simulink model "MIT_bus_ver3"  (Simulink 8.8)
settings: Solver=VariableStepAuto  StartTime=0.0  StopTime=10.0  RelTol=1e-3
libraries: powerlib x94
settings Model: Creator=jherna4  LastModifiedBy=jherna4
settings DataIOCC: LimitDataPoints=off  SaveFormat=Dataset  SignalLoggingSaveFormat=Dataset
settings DebuggingCC: UnderspecifiedInitializationDetection=Simplified  MergeDetectMultiDrivingBlocksExec=error  FcnCallInpInsideContextMsg=error  StateNameClashWarn=none  SFUnexpectedBacktrackingDiag=error  SFNoUnconditionalDefaultTransitionDiag=error
settings HardwareCC: ProdBitPerPointer=64  ProdBitPerSizeT=64  ProdBitPerPtrDiffT=64  ProdLargestAtomicFloat=Float  ProdIntDivRoundTo=Zero  ProdEndianess=LittleEndian  ProdWordSize=64  ProdHWDeviceType=Intel->x86-64 (Windows64)
settings ModelReferenceCC: PropagateSignalLabelsOutOfModel=on
settings GRTTargetCC: TargetLangStandard=C99 (ISO)  GeneratePreprocessorConditionals=Use local settings  CombineOutputUpdateFcns=on  GRTInterface=off
settings ConfigComp: CovMetricSettings=dwe  CovHtmlReporting=off  CovSaveCumulativeToWorkspaceVar=off  CovSaveSingleToWorkspaceVar=off  CovExternalEMLEnable=on

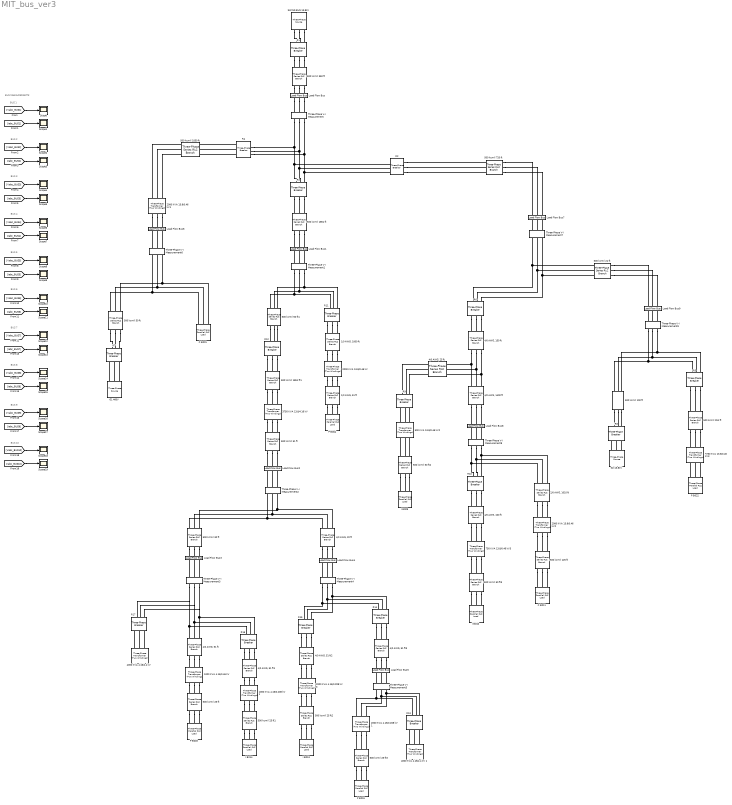
== system MIT_bus_ver3 ==
  note: BUS MEASUREMENTS:
  note: BUS 1
  note: BUS 2
  note: BUS 3
  note: BUS 4
  note: BUS 5
  note: BUS 6
  note: BUS 7
  note: BUS 8
  note: BUS 9
  note: BUS 10
  "1/0 AWG, 1000 ft" : powerlib/Elements/Three-Phase Series RLC Branch  LConnTagsString=A|B|C  RConnTagsString=A|B|C  BranchType=RL  Resistance=128e-3  Inductance=109.81e-6  Measurements=None
  "1/0 AWG, 51 ft" : powerlib/Elements/Three-Phase Series RLC Branch  LConnTagsString=A|B|C  RConnTagsString=A|B|C  BranchType=RL  Resistance=6.53e-3  Inductance=5.6e-6  Measurements=None
  1000 KVA 4.16/0.208 kV 1 : powerlib/Elements/Three-Phase Transformer (Two Windings)  Winding1Connection=Yg  Winding2Connection=Yg  CoreType=Three single-phase transformers  SetSaturation=off  Hysteresis=off  DataFile='hysteresis'  SetInitialFlux=off  Measurements=None  UNITS=pu  NominalPower=[ 1000e3 , 60 ]  Winding1=[4.16e3 0.011 0.02]  Winding2=[0.208e3 0 0]  Rm=500  Lm=500  L0=0.5  Saturation=[0 0;0.0024 1.2;1 1.52]  InitialFluxes=[0.8 -0.8 0.7]  MoreParameters=off  BreakLoop=off  DataType=off  TransfoNumber=1
  "1000 KVA 4.16/0.46 kV " : powerlib/Elements/Three-Phase Transformer (Two Windings)  Winding1Connection=Yg  Winding2Connection=Yg  CoreType=Three single-phase transformers  SetSaturation=off  Hysteresis=off  DataFile='hysteresis'  SetInitialFlux=off  Measurements=None  UNITS=pu  NominalPower=[ 1000e3 , 60 ]  Winding1=[4.16e3 0.011 0.02]  Winding2=[0.46e3 0 0]  Rm=500  Lm=500  L0=0.5  Saturation=[0 0;0.0024 1.2;1 1.52]  InitialFluxes=[0.8 -0.8 0.7]  MoreParameters=off  BreakLoop=off  DataType=off  TransfoNumber=1
  "2/0 AWG, 1010 ft" : powerlib/Elements/Three-Phase Series RLC Branch  LConnTagsString=A|B|C  RConnTagsString=A|B|C  BranchType=RL  Resistance=103e-3  Inductance=109e-6  Measurements=None
  2000 KVA 13.8/0.46 kV : powerlib/Elements/Three-Phase Transformer (Two Windings)  Winding1Connection=Yg  Winding2Connection=Yg  CoreType=Three single-phase transformers  SetSaturation=off  Hysteresis=off  DataFile='hysteresis'  SetInitialFlux=off  Measurements=None  UNITS=pu  NominalPower=[ 2000e3 , 60 ]  Winding1=[13.8e3 0.011 0.02]  Winding2=[0.46e3 0 0]  Rm=500  Lm=500  L0=0.5  Saturation=[0 0;0.0024 1.2;1 1.52]  InitialFluxes=[0.8 -0.8 0.7]  MoreParameters=off  BreakLoop=off  DataType=off  TransfoNumber=1
  2000 KVA 13.8/0.46 kV1 : powerlib/Elements/Three-Phase Transformer (Two Windings)  Winding1Connection=Yg  Winding2Connection=Yg  CoreType=Three single-phase transformers  SetSaturation=off  Hysteresis=off  DataFile='hysteresis'  SetInitialFlux=off  Measurements=None  UNITS=pu  NominalPower=[ 2000e3 , 60 ]  Winding1=[13.8e3 0.011 0.02]  Winding2=[460 0 0]  Rm=500  Lm=500  L0=0.5  Saturation=[0 0;0.0024 1.2;1 1.52]  InitialFluxes=[0.8 -0.8 0.7]  MoreParameters=off  BreakLoop=off  DataType=off  TransfoNumber=1
  2000 KVA 13.8/0.46 kV2 : powerlib/Elements/Three-Phase Transformer (Two Windings)  Winding1Connection=Yg  Winding2Connection=Yg  CoreType=Three single-phase transformers  SetSaturation=off  Hysteresis=off  DataFile='hysteresis'  SetInitialFlux=off  Measurements=None  UNITS=pu  NominalPower=[ 2000e3 , 60 ]  Winding1=[13.8e3 0.011 0.02]  Winding2=[0.46e3 0 0]  Rm=500  Lm=500  L0=0.5  Saturation=[0 0;0.0024 1.2;1 1.52]  InitialFluxes=[0.8 -0.8 0.7]  MoreParameters=off  BreakLoop=off  DataType=off  TransfoNumber=1
  2000 KVA 4.16/0.208 kV 1 : powerlib/Elements/Three-Phase Transformer (Two Windings)  Winding1Connection=Yg  Winding2Connection=Yg  CoreType=Three single-phase transformers  SetSaturation=off  Hysteresis=off  DataFile='hysteresis'  SetInitialFlux=off  Measurements=None  UNITS=pu  NominalPower=[ 2000e3 , 60 ]  Winding1=[4.16e3 0.011 0.02]  Winding2=[0.208e3 0 0]  Rm=500  Lm=500  L0=0.5  Saturation=[0 0;0.0024 1.2;1 1.52]  InitialFluxes=[0.8 -0.8 0.7]  MoreParameters=off  BreakLoop=off  DataType=off  TransfoNumber=1
  2000 KVA 4.16/0.208 kV 3 : powerlib/Elements/Three-Phase Transformer (Two Windings)  Winding1Connection=Yg  Winding2Connection=Yg  CoreType=Three single-phase transformers  SetSaturation=off  Hysteresis=off  DataFile='hysteresis'  SetInitialFlux=off  Measurements=None  UNITS=pu  NominalPower=[ 2000e3 , 60 ]  Winding1=[4.16e3 0.011 0.02]  Winding2=[0.208e3 0 0]  Rm=500  Lm=500  L0=0.5  Saturation=[0 0;0.0024 1.2;1 1.52]  InitialFluxes=[0.8 -0.8 0.7]  MoreParameters=off  BreakLoop=off  DataType=off  TransfoNumber=1
  3750 KVA 13.8/0.46 kV3 : powerlib/Elements/Three-Phase Transformer (Two Windings)  Winding1Connection=Yg  Winding2Connection=Yg  CoreType=Three single-phase transformers  SetSaturation=off  Hysteresis=off  DataFile='hysteresis'  SetInitialFlux=off  Measurements=None  UNITS=pu  NominalPower=[ 3750e3 , 60 ]  Winding1=[13.8e3 0.011 0.02]  Winding2=[0.46e3 0 0]  Rm=500  Lm=500  L0=0.5  Saturation=[0 0;0.0024 1.2;1 1.52]  InitialFluxes=[0.8 -0.8 0.7]  MoreParameters=off  BreakLoop=off  DataType=off  TransfoNumber=1
  "3750 KVA 13.8/4.16 kV " : powerlib/Elements/Three-Phase Transformer (Two Windings)  Winding1Connection=Yg  Winding2Connection=Yg  CoreType=Three single-phase transformers  SetSaturation=off  Hysteresis=off  DataFile='hysteresis'  SetInitialFlux=off  Measurements=None  UNITS=pu  NominalPower=[ 3750e3 , 60 ]  Winding1=[13.8e3 0.011 0.02]  Winding2=[4.16e3 0 0]  Rm=500  Lm=500  L0=0.5  Saturation=[0 0;0.0024 1.2;1 1.52]  InitialFluxes=[0.8 -0.8 0.7]  MoreParameters=off  BreakLoop=off  DataType=off  TransfoNumber=1
  "4/0 AWG, 100 ft" : powerlib/Elements/Three-Phase Series RLC Branch  LConnTagsString=A|B|C  RConnTagsString=A|B|C  BranchType=RL  Resistance=6.4e-3  Inductance=10.11e-6  Measurements=None
  "4/0 AWG, 1400 ft" : powerlib/Elements/Three-Phase Series RLC Branch  LConnTagsString=A|B|C  RConnTagsString=A|B|C  BranchType=RL  Resistance=89.6e-3  Inductance=141.5e-6  Measurements=None
  "4/0 AWG, 150 ft" : powerlib/Elements/Three-Phase Series RLC Branch  LConnTagsString=A|B|C  RConnTagsString=A|B|C  BranchType=RL  Resistance=9.6e-3  Inductance=15.16e-6  Measurements=None
  "4/0 AWG, 20 ft" : powerlib/Elements/Three-Phase Series RLC Branch  LConnTagsString=A|B|C  RConnTagsString=A|B|C  BranchType=RL  Resistance=1.28e-3  Inductance=2.02e-6  Measurements=None
  "4/0 AWG, 25 ft" : powerlib/Elements/Three-Phase Series RLC Branch  LConnTagsString=A|B|C  RConnTagsString=A|B|C  BranchType=RL  Resistance=1.6e-3  Inductance=2.53e-6  Measurements=None
  4/0 AWG, 51 ft{,1..3} (4 alike) : powerlib/Elements/Three-Phase Series RLC Branch  LConnTagsString=A|B|C  RConnTagsString=A|B|C  BranchType=RL  Resistance=3.264e-3  Inductance=5.15e-6  Measurements=None
  4000 KVA 4.16/2.4 kV : powerlib/Elements/Three-Phase Transformer (Two Windings)  Winding1Connection=Yg  Winding2Connection=Yg  CoreType=Three single-phase transformers  SetSaturation=off  Hysteresis=off  DataFile='hysteresis'  SetInitialFlux=off  Measurements=None  UNITS=pu  NominalPower=[ 4000e3 , 60 ]  Winding1=[4160 0.011 0.02]  Winding2=[2400 0 0]  Rm=500  Lm=500  L0=0.5  Saturation=[0 0;0.0024 1.2;1 1.52]  InitialFluxes=[0.8 -0.8 0.7]  MoreParameters=off  BreakLoop=off  DataType=off  TransfoNumber=1
  4000 KVA 4.16/2.4 kV 1 : powerlib/Elements/Three-Phase Transformer (Two Windings)  Winding1Connection=Yg  Winding2Connection=Yg  CoreType=Three single-phase transformers  SetSaturation=off  Hysteresis=off  DataFile='hysteresis'  SetInitialFlux=off  Measurements=None  UNITS=pu  NominalPower=[ 4000e3 , 60 ]  Winding1=[4.16e3 0.011 0.02]  Winding2=[2.4e3 0 0]  Rm=500  Lm=500  L0=0.5  Saturation=[0 0;0.0024 1.2;1 1.52]  InitialFluxes=[0.8 -0.8 0.7]  MoreParameters=off  BreakLoop=off  DataType=off  TransfoNumber=1
  500 KVA 13.8/0.46 kV2 : powerlib/Elements/Three-Phase Transformer (Two Windings)  Winding1Connection=Yg  Winding2Connection=Yg  CoreType=Three single-phase transformers  SetSaturation=off  Hysteresis=off  DataFile='hysteresis'  SetInitialFlux=off  Measurements=None  UNITS=pu  NominalPower=[ 500e3 , 60 ]  Winding1=[13.8e3 0.011 0.02]  Winding2=[0.46e3 0 0]  Rm=500  Lm=500  L0=0.5  Saturation=[0 0;0.0024 1.2;1 1.52]  InitialFluxes=[0.8 -0.8 0.7]  MoreParameters=off  BreakLoop=off  DataType=off  TransfoNumber=1
  500 kcmil 100 ft : powerlib/Elements/Three-Phase Series RLC Branch  LConnTagsString=A|B|C  RConnTagsString=A|B|C  BranchType=RL  Resistance=2.94e-3  Inductance=9.26e-6  Measurements=None
  500 kcmil 1050 ft : powerlib/Elements/Three-Phase Series RLC Branch  LConnTagsString=A|B|C  RConnTagsString=A|B|C  BranchType=RL  Resistance=30.87e-3  Inductance=97.2e-6  Measurements=None
  500 kcmil 125 ft : powerlib/Elements/Three-Phase Series RLC Branch  LConnTagsString=A|B|C  RConnTagsString=A|B|C  BranchType=RL  Resistance=3.7e-3  Inductance=11.6e-6  Measurements=None
  500 kcmil 1851 ft : powerlib/Elements/Three-Phase Series RLC Branch  LConnTagsString=A|B|C  RConnTagsString=A|B|C  BranchType=RL  Resistance=54.41e-3  Inductance=171.36e-6  Measurements=None
  500 kcmil 1851 ft1 : powerlib/Elements/Three-Phase Series RLC Branch  LConnTagsString=A|B|C  RConnTagsString=A|B|C  BranchType=RL  Resistance=54.41e-3  Inductance=171.36e-6  Measurements=None
  500 kcmil 21 ft : powerlib/Elements/Three-Phase Series RLC Branch  LConnTagsString=A|B|C  RConnTagsString=A|B|C  BranchType=RL  Resistance=0.62e-3  Inductance=1.94e-6  Measurements=None
  500 kcmil 25 ft{,1..3} (4 alike) : powerlib/Elements/Three-Phase Series RLC Branch  LConnTagsString=A|B|C  RConnTagsString=A|B|C  BranchType=RL  Resistance=0.735e-3  Inductance=2.31e-6  Measurements=None
  500 kcmil 251 ft : powerlib/Elements/Three-Phase Series RLC Branch  LConnTagsString=A|B|C  RConnTagsString=A|B|C  BranchType=RL  Resistance=7.38e-3  Inductance=23.24e-6  Measurements=None
  500 kcmil 30 ft : powerlib/Elements/Three-Phase Series RLC Branch  LConnTagsString=A|B|C  RConnTagsString=A|B|C  BranchType=RL  Resistance=0.88e-3  Inductance=2.78e-6  Measurements=None
  500 kcmil 350 ft : powerlib/Elements/Three-Phase Series RLC Branch  LConnTagsString=A|B|C  RConnTagsString=A|B|C  BranchType=RL  Resistance=10.29e-3  Inductance=32.4e-6  Measurements=None
  500 kcmil 50 ft{,1..3} (4 alike) : powerlib/Elements/Three-Phase Series RLC Branch  LConnTagsString=A|B|C  RConnTagsString=A|B|C  BranchType=RL  Resistance=1.47e-3  Inductance=4.63e-6  Measurements=None
  500 kcmil 51 ft : powerlib/Elements/Three-Phase Series RLC Branch  LConnTagsString=A|B|C  RConnTagsString=A|B|C  BranchType=RL  Resistance=1.5e-3  Inductance=4.72e-6  Measurements=None
  500 kcmil 720 ft : powerlib/Elements/Three-Phase Series RLC Branch  LConnTagsString=A|B|C  RConnTagsString=A|B|C  BranchType=RL  Resistance=21.17e-3  Inductance=66.65e-6  Measurements=None
  750 KVA 13.8/0.46 kV3 : powerlib/Elements/Three-Phase Transformer (Two Windings)  Winding1Connection=Yg  Winding2Connection=Yg  CoreType=Three single-phase transformers  SetSaturation=off  Hysteresis=off  DataFile='hysteresis'  SetInitialFlux=off  Measurements=None  UNITS=pu  NominalPower=[ 750e3 , 60 ]  Winding1=[13.8e3 0.011 0.02]  Winding2=[0.46e3 0 0]  Rm=500  Lm=500  L0=0.5  Saturation=[0 0;0.0024 1.2;1 1.52]  InitialFluxes=[0.8 -0.8 0.7]  MoreParameters=off  BreakLoop=off  DataType=off  TransfoNumber=1
  C B001 : powerlib/Elements/Three-Phase Parallel RLC Load  LConnTagsString=A|B|C  Configuration=Y (grounded)  NominalVoltage=460  Vabc=[1e3 1e3 1e3]  Vabcp=[1e3 1e3 1e3]  NominalFrequency=60  UnbalancedPower=off  ActivePower=10e3  InductivePower=100  CapacitivePower=100  Pabc=[10e3 9e3 11e3]  QLabc=[100 90 110]  QCabc=[100 90 110]  Pabcp=[10e3 9e3 11e3]  QLabcp=[100 90 110]  QCabcp=[100 90 110]  Measurements=None  LoadType=constant Z
  C B011 : powerlib/Elements/Three-Phase Parallel RLC Load  LConnTagsString=A|B|C  Configuration=Y (grounded)  NominalVoltage=460  Vabc=[1e3 1e3 1e3]  Vabcp=[1e3 1e3 1e3]  NominalFrequency=60  UnbalancedPower=off  ActivePower=10e3  InductivePower=100  CapacitivePower=100  Pabc=[10e3 9e3 11e3]  QLabc=[100 90 110]  QCabc=[100 90 110]  Pabcp=[10e3 9e3 11e3]  QLabcp=[100 90 110]  QCabcp=[100 90 110]  Measurements=None  LoadType=constant Z
  G1 460V : powerlib/Electrical Sources/Three-Phase Source  InternalConnection=Yg  VoltagePhases=on  Voltage=120e3  PhaseAngle=0  Voltage_phases=[1 1 1]*460/sqrt(3)  PhaseAngles_phases=[ 0 -120 120]  Frequency=60  NonIdealSource=off  SpecifyImpedance=on  Resistance=0.8929  Inductance=16.58e-3  ShortCircuitLevel=100e6  BaseVoltage=120e3  XRratio=10  BusType=swing  Pref=0  Qref=0  Prefabc=[0 0 0]  Qrefabc=[0 0 0]  Qmin="[-inf  -inf -inf]"  Qmax="[inf  inf inf]"
  G2 13.8kV : powerlib/Electrical Sources/Three-Phase Source  InternalConnection=Yg  VoltagePhases=on  Voltage=120e3  PhaseAngle=0  Voltage_phases=[1 1 1]*13.8e3/sqrt(3)  PhaseAngles_phases=[ 0 -120 120]  Frequency=60  NonIdealSource=off  SpecifyImpedance=on  Resistance=0.8929  Inductance=16.58e-3  ShortCircuitLevel=100e6  BaseVoltage=120e3  XRratio=10  BusType=swing  Pref=0  Qref=0  Prefabc=[0 0 0]  Qrefabc=[0 0 0]  Qmin="[-inf  -inf -inf]"  Qmax="[inf  inf inf]"
  I B009 : powerlib/Elements/Three-Phase Parallel RLC Load  LConnTagsString=A|B|C  Configuration=Y (grounded)  NominalVoltage=460  Vabc=[1e3 1e3 1e3]  Vabcp=[1e3 1e3 1e3]  NominalFrequency=60  UnbalancedPower=off  ActivePower=10e3  InductivePower=100  CapacitivePower=100  Pabc=[10e3 9e3 11e3]  QLabc=[100 90 110]  QCabc=[100 90 110]  Pabcp=[10e3 9e3 11e3]  QLabcp=[100 90 110]  QCabcp=[100 90 110]  Measurements=None  LoadType=constant Z
  I B010 : powerlib/Elements/Three-Phase Parallel RLC Load  LConnTagsString=A|B|C  Configuration=Y (grounded)  NominalVoltage=460  Vabc=[1e3 1e3 1e3]  Vabcp=[1e3 1e3 1e3]  NominalFrequency=60  UnbalancedPower=off  ActivePower=10e3  InductivePower=100  CapacitivePower=100  Pabc=[10e3 9e3 11e3]  QLabc=[100 90 110]  QCabc=[100 90 110]  Pabcp=[10e3 9e3 11e3]  QLabcp=[100 90 110]  QCabcp=[100 90 110]  Measurements=None  LoadType=constant Z
  I B013 : powerlib/Elements/Three-Phase Parallel RLC Load  LConnTagsString=A|B|C  Configuration=Y (grounded)  NominalVoltage=208  Vabc=[1e3 1e3 1e3]  Vabcp=[1e3 1e3 1e3]  NominalFrequency=60  UnbalancedPower=off  ActivePower=10e3  InductivePower=100  CapacitivePower=100  Pabc=[10e3 9e3 11e3]  QLabc=[100 90 110]  QCabc=[100 90 110]  Pabcp=[10e3 9e3 11e3]  QLabcp=[100 90 110]  QCabcp=[100 90 110]  Measurements=None  LoadType=constant Z
  I B014 : powerlib/Elements/Three-Phase Parallel RLC Load  LConnTagsString=A|B|C  Configuration=Y (grounded)  NominalVoltage=208  Vabc=[1e3 1e3 1e3]  Vabcp=[1e3 1e3 1e3]  NominalFrequency=60  UnbalancedPower=off  ActivePower=10e3  InductivePower=100  CapacitivePower=100  Pabc=[10e3 9e3 11e3]  QLabc=[100 90 110]  QCabc=[100 90 110]  Pabcp=[10e3 9e3 11e3]  QLabcp=[100 90 110]  QCabcp=[100 90 110]  Measurements=None  LoadType=constant Z
  Load Flow Bus : powerlib/Measurements/Load Flow Bus  LConnTagsString=a|b|c  RConnTagsString=a|b|c  Phases=ABC  Connectors=on both sides  ID=BUS1  Vbase=13.8e3/sqrt(3)  Vref=[1 1 1]  Vangle=[0 -120 120]  VLF=1  VLFb=1  VLFc=1  angleLF=0  angleLFb=0  angleLFc=0
  Load Flow Bus1 : powerlib/Measurements/Load Flow Bus  LConnTagsString=a|b|c  RConnTagsString=a|b|c  Phases=ABC  Connectors=on both sides  ID=BUS3  Vbase=13.8e3/sqrt(3)  Vref=[1 1 1]  Vangle=[1 -120 120]  VLF=1  VLFb=1  VLFc=1  angleLF=0  angleLFb=0  angleLFc=0
  Load Flow Bus2 : powerlib/Measurements/Load Flow Bus  LConnTagsString=a|b|c  RConnTagsString=a|b|c  Phases=ABC  Connectors=on both sides  ID=BUS4  Vbase=4.16e3/sqrt(3)  Vref=[1 1 1]  Vangle=[0 -120 120]  VLF=1  VLFb=1  VLFc=1  angleLF=0  angleLFb=0  angleLFc=0
  Load Flow Bus3 : powerlib/Measurements/Load Flow Bus  LConnTagsString=a|b|c  RConnTagsString=a|b|c  Phases=ABC  Connectors=on both sides  ID=BUS5  Vbase=4.16e3/sqrt(3)  Vref=[1 1 1]  Vangle=[0 -120 120]  VLF=1  VLFb=1  VLFc=1  angleLF=0  angleLFb=0  angleLFc=0
  Load Flow Bus4 : powerlib/Measurements/Load Flow Bus  LConnTagsString=a|b|c  RConnTagsString=a|b|c  Phases=ABC  Connectors=on both sides  ID=BUS6  Vbase=4.16e3/sqrt(3)  Vref=[1 1 1]  Vangle=[0 -120 120]  VLF=1  VLFb=1  VLFc=1  angleLF=0  angleLFb=0  angleLFc=0
  Load Flow Bus5 : powerlib/Measurements/Load Flow Bus  LConnTagsString=a|b|c  RConnTagsString=a|b|c  Phases=ABC  Connectors=on both sides  ID=BUS7  Vbase=4.16e3/sqrt(3)  Vref=[1 1 1]  Vangle=[0 -120 120]  VLF=1  VLFb=1  VLFc=1  angleLF=0  angleLFb=0  angleLFc=0
  Load Flow Bus6 : powerlib/Measurements/Load Flow Bus  LConnTagsString=a|b|c  RConnTagsString=a|b|c  Phases=ABC  Connectors=on both sides  ID=BUS2  Vbase=460/sqrt(3)  Vref=[1 1 1]  Vangle=[0 -120 120]  VLF=1  VLFb=1  VLFc=1  angleLF=0  angleLFb=0  angleLFc=0
  Load Flow Bus7 : powerlib/Measurements/Load Flow Bus  LConnTagsString=a|b|c  RConnTagsString=a|b|c  Phases=ABC  Connectors=on both sides  ID=BUS8  Vbase=13.8e3/sqrt(3)  Vref=[1 1 1]  Vangle=[0 -120 120]  VLF=1  VLFb=1  VLFc=1  angleLF=0  angleLFb=0  angleLFc=0
  Load Flow Bus8 : powerlib/Measurements/Load Flow Bus  LConnTagsString=a|b|c  RConnTagsString=a|b|c  Phases=ABC  Connectors=on both sides  ID=BUS9  Vbase=13.8e3/sqrt(3)  Vref=[1 1 1]  Vangle=[0 -120 120]  VLF=1  VLFb=1  VLFc=1  angleLF=0  angleLFb=0  angleLFc=0
  Load Flow Bus9 : powerlib/Measurements/Load Flow Bus  LConnTagsString=a|b|c  RConnTagsString=a|b|c  Phases=ABC  Connectors=on both sides  ID=BUS10  Vbase=13.8e3/sqrt(3)  Vref=[1 1 1]  Vangle=[0 -120 120]  VLF=1  VLFb=1  VLFc=1  angleLF=0  angleLFb=0  angleLFc=0
  P B003 : powerlib/Elements/Three-Phase Parallel RLC Load  LConnTagsString=A|B|C  Configuration=Y (grounded)  NominalVoltage=460  Vabc=[1e3 1e3 1e3]  Vabcp=[1e3 1e3 1e3]  NominalFrequency=60  UnbalancedPower=off  ActivePower=10e3  InductivePower=100  CapacitivePower=100  Pabc=[10e3 9e3 11e3]  QLabc=[100 90 110]  QCabc=[100 90 110]  Pabcp=[10e3 9e3 11e3]  QLabcp=[100 90 110]  QCabcp=[100 90 110]  Measurements=None  LoadType=constant Z
  P B004 : powerlib/Elements/Three-Phase Parallel RLC Load  LConnTagsString=A|B|C  Configuration=Y (grounded)  NominalVoltage=460  Vabc=[1e3 1e3 1e3]  Vabcp=[1e3 1e3 1e3]  NominalFrequency=60  UnbalancedPower=off  ActivePower=10e3  InductivePower=100  CapacitivePower=100  Pabc=[10e3 9e3 11e3]  QLabc=[100 90 110]  QCabc=[100 90 110]  Pabcp=[10e3 9e3 11e3]  QLabcp=[100 90 110]  QCabcp=[100 90 110]  Measurements=None  LoadType=constant Z
  P B015 : powerlib/Elements/Three-Phase Parallel RLC Load  LConnTagsString=A|B|C  Configuration=Y (grounded)  NominalVoltage=208  Vabc=[1e3 1e3 1e3]  Vabcp=[1e3 1e3 1e3]  NominalFrequency=60  UnbalancedPower=off  ActivePower=10e3  InductivePower=100  CapacitivePower=100  Pabc=[10e3 9e3 11e3]  QLabc=[100 90 110]  QCabc=[100 90 110]  Pabcp=[10e3 9e3 11e3]  QLabcp=[100 90 110]  QCabcp=[100 90 110]  Measurements=None  LoadType=constant Z
  P B022 : powerlib/Elements/Three-Phase Parallel RLC Load  LConnTagsString=A|B|C  Configuration=Y (grounded)  NominalVoltage=460  Vabc=[1e3 1e3 1e3]  Vabcp=[1e3 1e3 1e3]  NominalFrequency=60  UnbalancedPower=off  ActivePower=10e3  InductivePower=100  CapacitivePower=100  Pabc=[10e3 9e3 11e3]  QLabc=[100 90 110]  QCabc=[100 90 110]  Pabcp=[10e3 9e3 11e3]  QLabcp=[100 90 110]  QCabcp=[100 90 110]  Measurements=None  LoadType=constant Z
  R{1..17} (17 alike) : powerlib/Elements/Three-Phase Breaker  InitialState=closed  SwitchA=off  SwitchB=off  SwitchC=off  SwitchTimes=[0.5 ]  External=on  BreakerResistance=0.0001  SnubberResistance=inf  SnubberCapacitance=0  Measurements=None
  "SWING BUS 13.8kV " : powerlib/Electrical Sources/Three-Phase Source  InternalConnection=Yg  VoltagePhases=on  Voltage=120e3  PhaseAngle=0  Voltage_phases=[1 1 1]*13.8e3/sqrt(3)  PhaseAngles_phases=[ 0 -120 120]  Frequency=60  NonIdealSource=off  SpecifyImpedance=on  Resistance=0.8929  Inductance=16.58e-3  ShortCircuitLevel=100e6  BaseVoltage=120e3  XRratio=10  BusType=swing  Pref=0  Qref=0  Prefabc=[0 0 0]  Qrefabc=[0 0 0]  Qmin="[-inf  -inf -inf]"  Qmax="[inf  inf inf]"
  Scope{,1..19} (20 alike) : Scope
  Three-Phase V-I Measurement : powerlib/Measurements/Three-Phase V-I Measurement  VoltageMeasurement=phase-to-ground  SetLabelV=on  LabelV=Vabc_BUS1  Vpu=off  VpuLL=off  CurrentMeasurement=yes  SetLabelI=on  LabelI=Iabc_BUS1  Ipu=off  Pbase=100e6  Vbase=500e3  OutputType=Complex  PhasorSimulation=off  PSBequivalent=0
  Three-Phase V-I Measurement1 : powerlib/Measurements/Three-Phase V-I Measurement  VoltageMeasurement=phase-to-ground  SetLabelV=on  LabelV=Vabc_BUS3  Vpu=off  VpuLL=off  CurrentMeasurement=yes  SetLabelI=on  LabelI=Iabc_BUS3  Ipu=off  Pbase=100e6  Vbase=500e3  OutputType=Complex  PhasorSimulation=off  PSBequivalent=0
  Three-Phase V-I Measurement2 : powerlib/Measurements/Three-Phase V-I Measurement  VoltageMeasurement=phase-to-ground  SetLabelV=on  LabelV=Vabc_BUS4  Vpu=off  VpuLL=off  CurrentMeasurement=yes  SetLabelI=on  LabelI=Iabc_BUS4  Ipu=off  Pbase=100e6  Vbase=500e3  OutputType=Complex  PhasorSimulation=off  PSBequivalent=0
  Three-Phase V-I Measurement3 : powerlib/Measurements/Three-Phase V-I Measurement  VoltageMeasurement=phase-to-ground  SetLabelV=on  LabelV=Vabc_BUS5  Vpu=off  VpuLL=off  CurrentMeasurement=yes  SetLabelI=on  LabelI=Iabc_BUS5  Ipu=off  Pbase=100e6  Vbase=500e3  OutputType=Complex  PhasorSimulation=off  PSBequivalent=0
  Three-Phase V-I Measurement4 : powerlib/Measurements/Three-Phase V-I Measurement  VoltageMeasurement=phase-to-ground  SetLabelV=on  LabelV=Vabc_BUS6  Vpu=off  VpuLL=off  CurrentMeasurement=yes  SetLabelI=on  LabelI=Iabc_BUS6  Ipu=off  Pbase=100e6  Vbase=500e3  OutputType=Complex  PhasorSimulation=off  PSBequivalent=0
  Three-Phase V-I Measurement5 : powerlib/Measurements/Three-Phase V-I Measurement  VoltageMeasurement=phase-to-ground  SetLabelV=on  LabelV=Vabc_BUS7  Vpu=off  VpuLL=off  CurrentMeasurement=yes  SetLabelI=on  LabelI=Iabc_BUS7  Ipu=off  Pbase=100e6  Vbase=500e3  OutputType=Complex  PhasorSimulation=off  PSBequivalent=0
  Three-Phase V-I Measurement6 : powerlib/Measurements/Three-Phase V-I Measurement  VoltageMeasurement=phase-to-ground  SetLabelV=on  LabelV=Vabc_BUS2  Vpu=off  VpuLL=off  CurrentMeasurement=yes  SetLabelI=on  LabelI=Iabc_BUS2  Ipu=off  Pbase=100e6  Vbase=500e3  OutputType=Complex  PhasorSimulation=off  PSBequivalent=0
  Three-Phase V-I Measurement7 : powerlib/Measurements/Three-Phase V-I Measurement  VoltageMeasurement=phase-to-ground  SetLabelV=on  LabelV=Vabc_BUS8  Vpu=off  VpuLL=off  CurrentMeasurement=yes  SetLabelI=on  LabelI=Iabc_BUS8  Ipu=off  Pbase=100e6  Vbase=500e3  OutputType=Complex  PhasorSimulation=off  PSBequivalent=0
  Three-Phase V-I Measurement8 : powerlib/Measurements/Three-Phase V-I Measurement  VoltageMeasurement=phase-to-ground  SetLabelV=on  LabelV=Vabc_BUS9  Vpu=off  VpuLL=off  CurrentMeasurement=yes  SetLabelI=on  LabelI=Iabc_BUS9  Ipu=off  Pbase=100e6  Vbase=500e3  OutputType=Complex  PhasorSimulation=off  PSBequivalent=0
  Three-Phase V-I Measurement9 : powerlib/Measurements/Three-Phase V-I Measurement  VoltageMeasurement=phase-to-ground  SetLabelV=on  LabelV=Vabc_BUS10  Vpu=off  VpuLL=off  CurrentMeasurement=yes  SetLabelI=on  LabelI=Iabc_BUS10  Ipu=off  Pbase=100e6  Vbase=500e3  OutputType=Complex  PhasorSimulation=off  PSBequivalent=0
  wires:
  [Vabc_BUS1] -> Scope/1
  [Iabc_BUS1] -> Scope1/1
  [Vabc_BUS2] -> Scope2/1
  [Iabc_BUS2] -> Scope3/1
  [Vabc_BUS3] -> Scope4/1
  [Iabc_BUS3] -> Scope5/1
  [Vabc_BUS4] -> Scope6/1
  [Iabc_BUS4] -> Scope7/1
  [Vabc_BUS5] -> Scope8/1
  [Iabc_BUS5] -> Scope9/1
  [Vabc_BUS6] -> Scope10/1
  [Iabc_BUS6] -> Scope11/1
  [Vabc_BUS7] -> Scope12/1
  [Iabc_BUS7] -> Scope13/1
  [Vabc_BUS8] -> Scope14/1
  [Iabc_BUS8] -> Scope15/1
  [Vabc_BUS9] -> Scope16/1
  [Iabc_BUS9] -> Scope17/1
  [Vabc_BUS10] -> Scope18/1
  [Iabc_BUS10] -> Scope19/1
  connections:
  "SWING BUS 13.8kV "/RConn1 -- R1/LConn1
  "SWING BUS 13.8kV "/RConn2 -- R1/LConn2
  "SWING BUS 13.8kV "/RConn3 -- R1/LConn3
  Three-Phase V-I Measurement1/RConn1 -- 500 kcmil 50 ft1/LConn1 -- R11/LConn1
  Three-Phase V-I Measurement1/RConn2 -- 500 kcmil 50 ft1/LConn2 -- R11/LConn2
  Three-Phase V-I Measurement1/RConn3 -- 500 kcmil 50 ft1/LConn3 -- R11/LConn3
  Load Flow Bus/RConn3 -- Three-Phase V-I Measurement/LConn3
  Load Flow Bus/RConn2 -- Three-Phase V-I Measurement/LConn2
  Load Flow Bus/RConn1 -- Three-Phase V-I Measurement/LConn1
  Three-Phase V-I Measurement/RConn3 -- R4/LConn3 -- R2/LConn3 -- R3/LConn3
  Three-Phase V-I Measurement/RConn2 -- R4/LConn2 -- R2/LConn2 -- R3/LConn2
  Three-Phase V-I Measurement/RConn1 -- R4/LConn1 -- R2/LConn1 -- R3/LConn1
  Three-Phase V-I Measurement1/LConn1 -- Load Flow Bus1/RConn1
  Three-Phase V-I Measurement1/LConn2 -- Load Flow Bus1/RConn2
  Three-Phase V-I Measurement1/LConn3 -- Load Flow Bus1/RConn3
  Three-Phase V-I Measurement2/LConn3 -- Load Flow Bus2/RConn3
  Three-Phase V-I Measurement2/LConn2 -- Load Flow Bus2/RConn2
  Three-Phase V-I Measurement2/LConn1 -- Load Flow Bus2/RConn1
  Three-Phase V-I Measurement3/RConn3 -- R17/LConn3 -- "4/0 AWG, 51 ft"/LConn3 -- R16/LConn3
  Three-Phase V-I Measurement3/RConn2 -- R17/LConn2 -- "4/0 AWG, 51 ft"/LConn2 -- R16/LConn2
  500 kcmil 30 ft/LConn1 -- "4/0 AWG, 20 ft"/LConn1 -- Three-Phase V-I Measurement2/RConn1
  4000 KVA 4.16/2.4 kV/LConn3 -- R17/RConn3
  4000 KVA 4.16/2.4 kV/LConn2 -- R17/RConn2
  4000 KVA 4.16/2.4 kV/LConn1 -- R17/RConn1
  Three-Phase V-I Measurement5/LConn2 -- Load Flow Bus5/RConn2
  Three-Phase V-I Measurement5/LConn1 -- Load Flow Bus5/RConn1
  Three-Phase V-I Measurement5/LConn3 -- Load Flow Bus5/RConn3
  2000 KVA 4.16/0.208 kV 1/LConn1 -- R13/LConn1 -- Three-Phase V-I Measurement5/RConn1
  2000 KVA 4.16/0.208 kV 1/LConn2 -- R13/LConn2 -- Three-Phase V-I Measurement5/RConn2
  2000 KVA 4.16/0.208 kV 1/LConn3 -- R13/LConn3 -- Three-Phase V-I Measurement5/RConn3
  4000 KVA 4.16/2.4 kV 1/LConn1 -- R13/RConn1
  4000 KVA 4.16/2.4 kV 1/LConn2 -- R13/RConn2
  4000 KVA 4.16/2.4 kV 1/LConn3 -- R13/RConn3
  500 kcmil 1050 ft/RConn3 -- 2000 KVA 13.8/0.46 kV1/LConn3
  500 kcmil 1050 ft/RConn2 -- 2000 KVA 13.8/0.46 kV1/LConn2
  500 kcmil 1050 ft/RConn1 -- 2000 KVA 13.8/0.46 kV1/LConn1
  2000 KVA 13.8/0.46 kV1/RConn3 -- Load Flow Bus6/LConn3
  2000 KVA 13.8/0.46 kV1/RConn2 -- Load Flow Bus6/LConn2
  2000 KVA 13.8/0.46 kV1/RConn1 -- Load Flow Bus6/LConn1
  Three-Phase V-I Measurement6/LConn1 -- Load Flow Bus6/RConn1
  Three-Phase V-I Measurement6/LConn2 -- Load Flow Bus6/RConn2
  Three-Phase V-I Measurement6/LConn3 -- Load Flow Bus6/RConn3
  C B001/LConn1 -- 500 kcmil 50 ft/LConn1 -- Three-Phase V-I Measurement6/RConn1
  C B001/LConn2 -- 500 kcmil 50 ft/LConn2 -- Three-Phase V-I Measurement6/RConn2
  C B001/LConn3 -- 500 kcmil 50 ft/LConn3 -- Three-Phase V-I Measurement6/RConn3
  Three-Phase V-I Measurement7/LConn1 -- Load Flow Bus7/RConn1
  Three-Phase V-I Measurement7/LConn3 -- Load Flow Bus7/RConn3
  Three-Phase V-I Measurement7/LConn2 -- Load Flow Bus7/RConn2
  500 KVA 13.8/0.46 kV2/LConn3 -- R9/RConn3
  500 KVA 13.8/0.46 kV2/LConn2 -- R9/RConn2
  500 KVA 13.8/0.46 kV2/LConn1 -- R9/RConn1
  Three-Phase V-I Measurement8/RConn3 -- "2/0 AWG, 1010 ft"/LConn3 -- R10/LConn3
  "4/0 AWG, 150 ft"/RConn1 -- "4/0 AWG, 1400 ft"/LConn1 -- "4/0 AWG, 25 ft"/LConn1
  "4/0 AWG, 150 ft"/RConn2 -- "4/0 AWG, 1400 ft"/LConn2 -- "4/0 AWG, 25 ft"/LConn2
  Three-Phase V-I Measurement9/RConn1 -- 500 kcmil 100 ft/LConn1 -- R5/LConn1
  Three-Phase V-I Measurement9/RConn2 -- 500 kcmil 100 ft/LConn2 -- R5/LConn2
  Three-Phase V-I Measurement9/RConn3 -- 500 kcmil 100 ft/LConn3 -- R5/LConn3
  G1 460V/RConn1 -- R7/RConn1
  G1 460V/RConn2 -- R7/RConn2
  G1 460V/RConn3 -- R7/RConn3
  Three-Phase V-I Measurement3/LConn1 -- Load Flow Bus3/RConn1
  Three-Phase V-I Measurement3/LConn3 -- Load Flow Bus3/RConn3
  Three-Phase V-I Measurement3/LConn2 -- Load Flow Bus3/RConn2
  500 kcmil 30 ft/LConn3 -- "4/0 AWG, 20 ft"/LConn3 -- Three-Phase V-I Measurement2/RConn3
  500 kcmil 30 ft/LConn2 -- "4/0 AWG, 20 ft"/LConn2 -- Three-Phase V-I Measurement2/RConn2
  Three-Phase V-I Measurement3/RConn1 -- R17/LConn1 -- "4/0 AWG, 51 ft"/LConn1 -- R16/LConn1
  Three-Phase V-I Measurement4/LConn3 -- Load Flow Bus4/RConn3
  Three-Phase V-I Measurement4/LConn2 -- Load Flow Bus4/RConn2
  Three-Phase V-I Measurement4/LConn1 -- Load Flow Bus4/RConn1
  R14/LConn1 -- Three-Phase V-I Measurement4/RConn1 -- R15/LConn1
  R14/LConn2 -- Three-Phase V-I Measurement4/RConn2 -- R15/LConn2
  R14/LConn3 -- Three-Phase V-I Measurement4/RConn3 -- R15/LConn3
  Three-Phase V-I Measurement8/LConn3 -- Load Flow Bus8/RConn3
  Three-Phase V-I Measurement8/LConn1 -- Load Flow Bus8/RConn1
  Three-Phase V-I Measurement8/LConn2 -- Load Flow Bus8/RConn2
  "4/0 AWG, 150 ft"/RConn3 -- "4/0 AWG, 1400 ft"/LConn3 -- "4/0 AWG, 25 ft"/LConn3
  Three-Phase V-I Measurement8/RConn2 -- "2/0 AWG, 1010 ft"/LConn2 -- R10/LConn2
  Three-Phase V-I Measurement8/RConn1 -- "2/0 AWG, 1010 ft"/LConn1 -- R10/LConn1
  Three-Phase V-I Measurement9/LConn3 -- Load Flow Bus9/RConn3
  Three-Phase V-I Measurement9/LConn1 -- Load Flow Bus9/RConn1
  Three-Phase V-I Measurement9/LConn2 -- Load Flow Bus9/RConn2
  R6/LConn1 -- 500 kcmil 21 ft/LConn1 -- Three-Phase V-I Measurement7/RConn1
  R6/LConn2 -- 500 kcmil 21 ft/LConn2 -- Three-Phase V-I Measurement7/RConn2
  R6/LConn3 -- 500 kcmil 21 ft/LConn3 -- Three-Phase V-I Measurement7/RConn3
  P B022/LConn3 -- 3750 KVA 13.8/0.46 kV3/RConn3
  P B022/LConn2 -- 3750 KVA 13.8/0.46 kV3/RConn2
  P B022/LConn1 -- 3750 KVA 13.8/0.46 kV3/RConn1
  G2 13.8kV/RConn3 -- R8/RConn3
  G2 13.8kV/RConn2 -- R8/RConn2
  G2 13.8kV/RConn1 -- R8/RConn1
  R1/RConn3 -- 500 kcmil 350 ft/LConn3
  R1/RConn2 -- 500 kcmil 350 ft/LConn2
  R1/RConn1 -- 500 kcmil 350 ft/LConn1
  500 kcmil 350 ft/RConn1 -- Load Flow Bus/LConn1
  500 kcmil 350 ft/RConn2 -- Load Flow Bus/LConn2
  500 kcmil 350 ft/RConn3 -- Load Flow Bus/LConn3
  500 kcmil 50 ft/RConn1 -- R7/LConn1
  500 kcmil 50 ft/RConn2 -- R7/LConn2
  500 kcmil 50 ft/RConn3 -- R7/LConn3
  R3/RConn3 -- 500 kcmil 1851 ft/LConn3
  500 kcmil 1851 ft/RConn3 -- Load Flow Bus1/LConn3
  R3/RConn2 -- 500 kcmil 1851 ft/LConn2
  500 kcmil 1851 ft/RConn2 -- Load Flow Bus1/LConn2
  R3/RConn1 -- 500 kcmil 1851 ft/LConn1
  500 kcmil 1851 ft/RConn1 -- Load Flow Bus1/LConn1
  500 kcmil 50 ft1/RConn3 -- R12/LConn3
  500 kcmil 50 ft1/RConn2 -- R12/LConn2
  500 kcmil 50 ft1/RConn1 -- R12/LConn1
  R12/RConn3 -- 500 kcmil 1851 ft1/LConn3
  500 kcmil 1851 ft1/RConn3 -- "3750 KVA 13.8/4.16 kV "/LConn3
  R12/RConn2 -- 500 kcmil 1851 ft1/LConn2
  500 kcmil 1851 ft1/RConn2 -- "3750 KVA 13.8/4.16 kV "/LConn2
  R12/RConn1 -- 500 kcmil 1851 ft1/LConn1
  500 kcmil 1851 ft1/RConn1 -- "3750 KVA 13.8/4.16 kV "/LConn1
  "3750 KVA 13.8/4.16 kV "/RConn3 -- 500 kcmil 51 ft/LConn3
  "3750 KVA 13.8/4.16 kV "/RConn2 -- 500 kcmil 51 ft/LConn2
  "3750 KVA 13.8/4.16 kV "/RConn1 -- 500 kcmil 51 ft/LConn1
  500 kcmil 51 ft/RConn3 -- Load Flow Bus2/LConn3
  500 kcmil 51 ft/RConn2 -- Load Flow Bus2/LConn2
  500 kcmil 51 ft/RConn1 -- Load Flow Bus2/LConn1
  R11/RConn1 -- "1/0 AWG, 1000 ft"/LConn1
  R11/RConn2 -- "1/0 AWG, 1000 ft"/LConn2
  R11/RConn3 -- "1/0 AWG, 1000 ft"/LConn3
  "1/0 AWG, 1000 ft"/RConn1 -- 2000 KVA 13.8/0.46 kV/LConn1
  "1/0 AWG, 1000 ft"/RConn2 -- 2000 KVA 13.8/0.46 kV/LConn2
  "1/0 AWG, 1000 ft"/RConn3 -- 2000 KVA 13.8/0.46 kV/LConn3
  2000 KVA 13.8/0.46 kV/RConn1 -- "1/0 AWG, 51 ft"/LConn1
  2000 KVA 13.8/0.46 kV/RConn2 -- "1/0 AWG, 51 ft"/LConn2
  2000 KVA 13.8/0.46 kV/RConn3 -- "1/0 AWG, 51 ft"/LConn3
  "1/0 AWG, 51 ft"/RConn1 -- P B004/LConn1
  "1/0 AWG, 51 ft"/RConn2 -- P B004/LConn2
  "1/0 AWG, 51 ft"/RConn3 -- P B004/LConn3
  500 kcmil 30 ft/RConn3 -- Load Flow Bus3/LConn3
  500 kcmil 30 ft/RConn2 -- Load Flow Bus3/LConn2
  500 kcmil 30 ft/RConn1 -- Load Flow Bus3/LConn1
  "4/0 AWG, 20 ft"/RConn3 -- Load Flow Bus4/LConn3
  "4/0 AWG, 20 ft"/RConn2 -- Load Flow Bus4/LConn2
  "4/0 AWG, 20 ft"/RConn1 -- Load Flow Bus4/LConn1
  "4/0 AWG, 51 ft"/RConn3 -- "1000 KVA 4.16/0.46 kV "/LConn3
  "4/0 AWG, 51 ft"/RConn2 -- "1000 KVA 4.16/0.46 kV "/LConn2
  "4/0 AWG, 51 ft"/RConn1 -- "1000 KVA 4.16/0.46 kV "/LConn1
  "1000 KVA 4.16/0.46 kV "/RConn3 -- 500 kcmil 25 ft/LConn3
  "1000 KVA 4.16/0.46 kV "/RConn2 -- 500 kcmil 25 ft/LConn2
  "1000 KVA 4.16/0.46 kV "/RConn1 -- 500 kcmil 25 ft/LConn1
  500 kcmil 25 ft/RConn1 -- P B003/LConn1
  500 kcmil 25 ft/RConn2 -- P B003/LConn2
  500 kcmil 25 ft/RConn3 -- P B003/LConn3
  R16/RConn3 -- "4/0 AWG, 51 ft1"/LConn3
  R16/RConn2 -- "4/0 AWG, 51 ft1"/LConn2
  R16/RConn1 -- "4/0 AWG, 51 ft1"/LConn1
  "4/0 AWG, 51 ft1"/RConn3 -- 1000 KVA 4.16/0.208 kV 1/LConn3
  "4/0 AWG, 51 ft1"/RConn2 -- 1000 KVA 4.16/0.208 kV 1/LConn2
  "4/0 AWG, 51 ft1"/RConn1 -- 1000 KVA 4.16/0.208 kV 1/LConn1
  1000 KVA 4.16/0.208 kV 1/RConn3 -- 500 kcmil 25 ft1/LConn3
  1000 KVA 4.16/0.208 kV 1/RConn2 -- 500 kcmil 25 ft1/LConn2
  1000 KVA 4.16/0.208 kV 1/RConn1 -- 500 kcmil 25 ft1/LConn1
  500 kcmil 25 ft1/RConn3 -- I B014/LConn3
  500 kcmil 25 ft1/RConn2 -- I B014/LConn2
  500 kcmil 25 ft1/RConn1 -- I B014/LConn1
  R15/RConn3 -- "4/0 AWG, 51 ft2"/LConn3
  R15/RConn2 -- "4/0 AWG, 51 ft2"/LConn2
  R15/RConn1 -- "4/0 AWG, 51 ft2"/LConn1
  "4/0 AWG, 51 ft2"/RConn3 -- 2000 KVA 4.16/0.208 kV 3/LConn3
  "4/0 AWG, 51 ft2"/RConn2 -- 2000 KVA 4.16/0.208 kV 3/LConn2
  "4/0 AWG, 51 ft2"/RConn1 -- 2000 KVA 4.16/0.208 kV 3/LConn1
  2000 KVA 4.16/0.208 kV 3/RConn3 -- 500 kcmil 25 ft2/LConn3
  2000 KVA 4.16/0.208 kV 3/RConn2 -- 500 kcmil 25 ft2/LConn2
  2000 KVA 4.16/0.208 kV 3/RConn1 -- 500 kcmil 25 ft2/LConn1
  500 kcmil 25 ft2/RConn1 -- I B013/LConn1
  500 kcmil 25 ft2/RConn2 -- I B013/LConn2
  500 kcmil 25 ft2/RConn3 -- I B013/LConn3
  R14/RConn1 -- "4/0 AWG, 51 ft3"/LConn1
  R14/RConn2 -- "4/0 AWG, 51 ft3"/LConn2
  R14/RConn3 -- "4/0 AWG, 51 ft3"/LConn3
  "4/0 AWG, 51 ft3"/RConn3 -- Load Flow Bus5/LConn3
  "4/0 AWG, 51 ft3"/RConn2 -- Load Flow Bus5/LConn2
  "4/0 AWG, 51 ft3"/RConn1 -- Load Flow Bus5/LConn1
  2000 KVA 4.16/0.208 kV 1/RConn3 -- 500 kcmil 25 ft3/LConn3
  2000 KVA 4.16/0.208 kV 1/RConn2 -- 500 kcmil 25 ft3/LConn2
  2000 KVA 4.16/0.208 kV 1/RConn1 -- 500 kcmil 25 ft3/LConn1
  500 kcmil 25 ft3/RConn3 -- P B015/LConn3
  500 kcmil 25 ft3/RConn2 -- P B015/LConn2
  500 kcmil 25 ft3/RConn1 -- P B015/LConn1
  500 kcmil 720 ft/RConn1 -- Load Flow Bus7/LConn1
  500 kcmil 720 ft/RConn2 -- Load Flow Bus7/LConn2
  500 kcmil 720 ft/RConn3 -- Load Flow Bus7/LConn3
  R2/RConn1 -- 500 kcmil 720 ft/LConn1
  R2/RConn2 -- 500 kcmil 720 ft/LConn2
  R2/RConn3 -- 500 kcmil 720 ft/LConn3
  R4/RConn1 -- 500 kcmil 1050 ft/LConn1
  R4/RConn2 -- 500 kcmil 1050 ft/LConn2
  R4/RConn3 -- 500 kcmil 1050 ft/LConn3
  R6/RConn1 -- "4/0 AWG, 150 ft"/LConn1
  R6/RConn2 -- "4/0 AWG, 150 ft"/LConn2
  R6/RConn3 -- "4/0 AWG, 150 ft"/LConn3
  "4/0 AWG, 25 ft"/RConn1 -- R9/LConn1
  "4/0 AWG, 25 ft"/RConn2 -- R9/LConn2
  "4/0 AWG, 25 ft"/RConn3 -- R9/LConn3
  "4/0 AWG, 1400 ft"/RConn1 -- Load Flow Bus8/LConn1
  "4/0 AWG, 1400 ft"/RConn2 -- Load Flow Bus8/LConn2
  "4/0 AWG, 1400 ft"/RConn3 -- Load Flow Bus8/LConn3
  500 kcmil 50 ft2/LConn3 -- 500 KVA 13.8/0.46 kV2/RConn3
  500 kcmil 50 ft2/LConn2 -- 500 KVA 13.8/0.46 kV2/RConn2
  500 kcmil 50 ft2/LConn1 -- 500 KVA 13.8/0.46 kV2/RConn1
  500 kcmil 50 ft2/RConn1 -- I B009/LConn1
  500 kcmil 50 ft2/RConn2 -- I B009/LConn2
  500 kcmil 50 ft2/RConn3 -- I B009/LConn3
  750 KVA 13.8/0.46 kV3/RConn3 -- 500 kcmil 50 ft3/LConn3
  750 KVA 13.8/0.46 kV3/RConn2 -- 500 kcmil 50 ft3/LConn2
  750 KVA 13.8/0.46 kV3/RConn1 -- 500 kcmil 50 ft3/LConn1
  500 kcmil 50 ft3/RConn1 -- I B010/LConn1
  500 kcmil 50 ft3/RConn2 -- I B010/LConn2
  500 kcmil 50 ft3/RConn3 -- I B010/LConn3
  R10/RConn1 -- "4/0 AWG, 100 ft"/LConn1
  R10/RConn2 -- "4/0 AWG, 100 ft"/LConn2
  R10/RConn3 -- "4/0 AWG, 100 ft"/LConn3
  "4/0 AWG, 100 ft"/RConn1 -- 750 KVA 13.8/0.46 kV3/LConn1
  "4/0 AWG, 100 ft"/RConn2 -- 750 KVA 13.8/0.46 kV3/LConn2
  "4/0 AWG, 100 ft"/RConn3 -- 750 KVA 13.8/0.46 kV3/LConn3
  "2/0 AWG, 1010 ft"/RConn1 -- 2000 KVA 13.8/0.46 kV2/LConn1
  "2/0 AWG, 1010 ft"/RConn2 -- 2000 KVA 13.8/0.46 kV2/LConn2
  "2/0 AWG, 1010 ft"/RConn3 -- 2000 KVA 13.8/0.46 kV2/LConn3
  2000 KVA 13.8/0.46 kV2/RConn1 -- 500 kcmil 125 ft/LConn1
  2000 KVA 13.8/0.46 kV2/RConn2 -- 500 kcmil 125 ft/LConn2
  2000 KVA 13.8/0.46 kV2/RConn3 -- 500 kcmil 125 ft/LConn3
  500 kcmil 125 ft/RConn1 -- C B011/LConn1
  500 kcmil 125 ft/RConn2 -- C B011/LConn2
  500 kcmil 125 ft/RConn3 -- C B011/LConn3
  500 kcmil 21 ft/RConn1 -- Load Flow Bus9/LConn1
  500 kcmil 21 ft/RConn2 -- Load Flow Bus9/LConn2
  500 kcmil 21 ft/RConn3 -- Load Flow Bus9/LConn3
  R5/RConn1 -- 500 kcmil 251 ft/LConn1
  R5/RConn2 -- 500 kcmil 251 ft/LConn2
  R5/RConn3 -- 500 kcmil 251 ft/LConn3
  500 kcmil 251 ft/RConn1 -- 3750 KVA 13.8/0.46 kV3/LConn1
  500 kcmil 251 ft/RConn2 -- 3750 KVA 13.8/0.46 kV3/LConn2
  500 kcmil 251 ft/RConn3 -- 3750 KVA 13.8/0.46 kV3/LConn3
  500 kcmil 100 ft/RConn1 -- R8/LConn1
  500 kcmil 100 ft/RConn2 -- R8/LConn2
  500 kcmil 100 ft/RConn3 -- R8/LConn3
